simulink model "TST_RmtAPP_DD2"  (R2016b)
settings: Solver=FixedStepDiscrete  StartTime=0.0  StopTime=simTime  FixedStep=sampleTime  RelTol=1e-3
values from neighbouring files (symbols this model uses):
  testCase = 1    [initTST_RmtAPP_DD2_001.m]    (also in initTST_RmtAPP_DD2_002.m = 2)
libraries: simulink x13, UnitTest_Lib x10
settings Model: Creator=bianxuyin  LastModifiedBy=bianxuyin
settings DebuggingCC: SignalRangeChecking=error

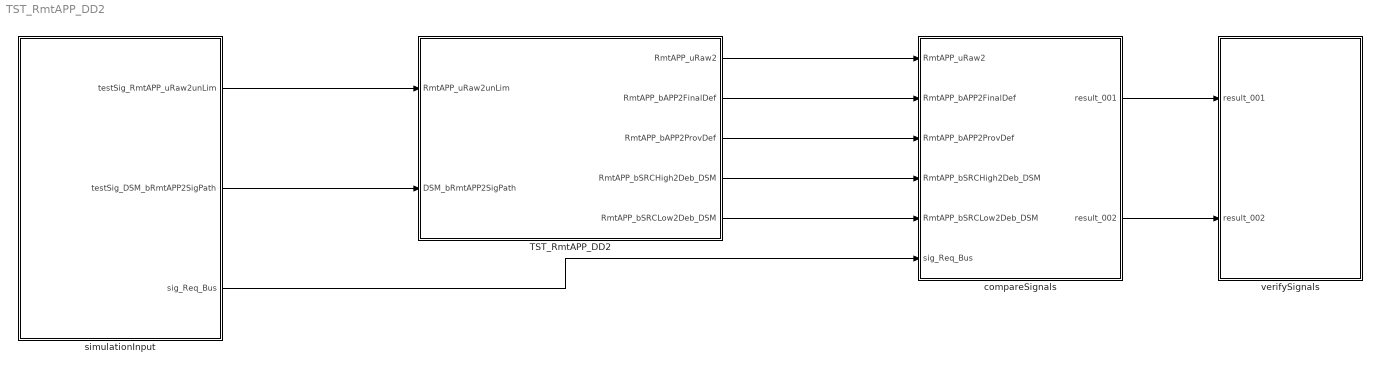
== system TST_RmtAPP_DD2 ==
  TST_RmtAPP_DD2 : Subsystem
  compareSignals : Subsystem
  simulationInput : Subsystem
  verifySignals : Subsystem
  wires:
  simulationInput/1(testSig_RmtAPP_uRaw2unLim) -> TST_RmtAPP_DD2/1(RmtAPP_uRaw2unLim)
  simulationInput/2(testSig_DSM_bRmtAPP2SigPath) -> TST_RmtAPP_DD2/2(DSM_bRmtAPP2SigPath)
  TST_RmtAPP_DD2/1(RmtAPP_uRaw2) -> compareSignals/1(RmtAPP_uRaw2)
  TST_RmtAPP_DD2/2(RmtAPP_bAPP2FinalDef) -> compareSignals/2(RmtAPP_bAPP2FinalDef)
  TST_RmtAPP_DD2/3(RmtAPP_bAPP2ProvDef) -> compareSignals/3(RmtAPP_bAPP2ProvDef)
  TST_RmtAPP_DD2/4(RmtAPP_bSRCHigh2Deb_DSM) -> compareSignals/4(RmtAPP_bSRCHigh2Deb_DSM)
  TST_RmtAPP_DD2/5(RmtAPP_bSRCLow2Deb_DSM) -> compareSignals/5(RmtAPP_bSRCLow2Deb_DSM)
  simulationInput/3(sig_Req_Bus) -> compareSignals/6(sig_Req_Bus)
  compareSignals/1(result_001) -> verifySignals/1(result_001)
  compareSignals/2(result_002) -> verifySignals/2(result_002)

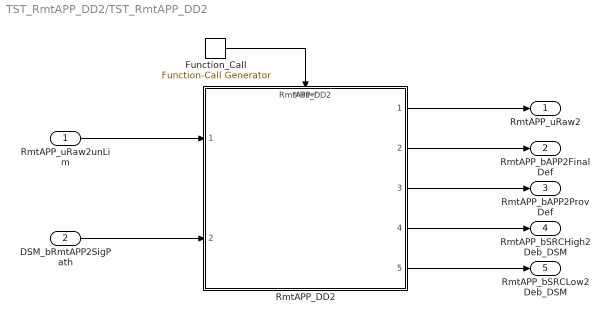
== system TST_RmtAPP_DD2/TST_RmtAPP_DD2 ==
  RmtAPP_uRaw2unLim : Inport
  DSM_bRmtAPP2SigPath : Inport  Port=2
  Function_Call : simulink/Ports & Subsystems/Function-Call Generator  sample_time=sampleTime  numberOfIterations=1
  RmtAPP_DD2 : ModelReference  ModelNameDialog=RmtAPP_DD2  SimulationMode=Normal  ModelReferenceVersion=1.5  TriggerPortName=function  TriggerPortTriggerType=function-call  TriggerPortStatesWhenEnabling=held
  RmtAPP_uRaw2 : Outport
  RmtAPP_bAPP2FinalDef : Outport  Port=2
  RmtAPP_bAPP2ProvDef : Outport  Port=3
  RmtAPP_bSRCHigh2Deb_DSM : Outport  Port=4
  RmtAPP_bSRCLow2Deb_DSM : Outport  Port=5
  wires:
  Function_Call/1 -> RmtAPP_DD2/Trigger
  RmtAPP_uRaw2unLim/1 -> RmtAPP_DD2/1
  DSM_bRmtAPP2SigPath/1 -> RmtAPP_DD2/2
  RmtAPP_DD2/1 -> RmtAPP_uRaw2/1
  RmtAPP_DD2/2 -> RmtAPP_bAPP2FinalDef/1
  RmtAPP_DD2/3 -> RmtAPP_bAPP2ProvDef/1
  RmtAPP_DD2/4 -> RmtAPP_bSRCHigh2Deb_DSM/1
  RmtAPP_DD2/5 -> RmtAPP_bSRCLow2Deb_DSM/1

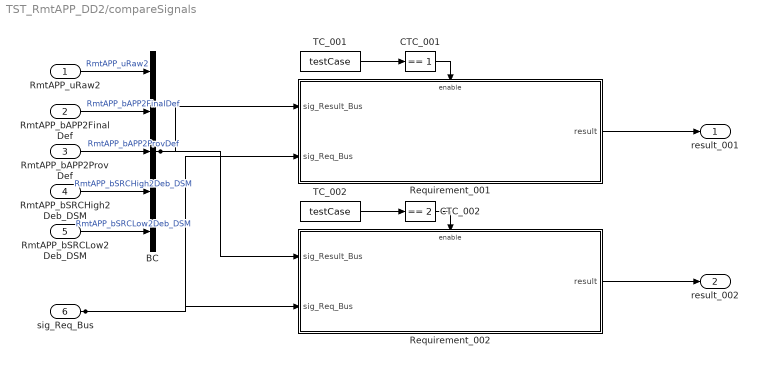
== system TST_RmtAPP_DD2/compareSignals ==
  RmtAPP_uRaw2 : Inport
  RmtAPP_bAPP2FinalDef : Inport  Port=2
  RmtAPP_bAPP2ProvDef : Inport  Port=3
  RmtAPP_bSRCHigh2Deb_DSM : Inport  Port=4
  RmtAPP_bSRCLow2Deb_DSM : Inport  Port=5
  sig_Req_Bus : Inport  Port=6
  BC : BusCreator  Inputs=5
  CTC_001 : simulink/Logic and Bit Operations/Compare To Constant  relop===  const=1  OutDataTypeStr=boolean
  CTC_002 : simulink/Logic and Bit Operations/Compare To Constant  relop===  const=2  OutDataTypeStr=boolean
  Requirement_001 : Subsystem
  Requirement_002 : Subsystem
  TC_001 : Constant  Value=testCase
  TC_002 : Constant  Value=testCase
  result_001 : Outport
  result_002 : Outport  Port=2
  wires:
  RmtAPP_uRaw2/1 -> BC/1  "RmtAPP_uRaw2"
  RmtAPP_bAPP2FinalDef/1 -> BC/2  "RmtAPP_bAPP2FinalDef"
  RmtAPP_bAPP2ProvDef/1 -> BC/3  "RmtAPP_bAPP2ProvDef"
  RmtAPP_bSRCHigh2Deb_DSM/1 -> BC/4  "RmtAPP_bSRCHigh2Deb_DSM"
  RmtAPP_bSRCLow2Deb_DSM/1 -> BC/5  "RmtAPP_bSRCLow2Deb_DSM"
  TC_001/1 -> CTC_001/1
  CTC_001/1 -> Requirement_001/Enable
  sig_Req_Bus/1 -> Requirement_001/2(sig_Req_Bus), Requirement_002/2(sig_Req_Bus)
  BC/1 -> Requirement_001/1(sig_Result_Bus), Requirement_002/1(sig_Result_Bus)
  Requirement_001/1(result) -> result_001/1
  TC_002/1 -> CTC_002/1
  CTC_002/1 -> Requirement_002/Enable
  Requirement_002/1(result) -> result_002/1

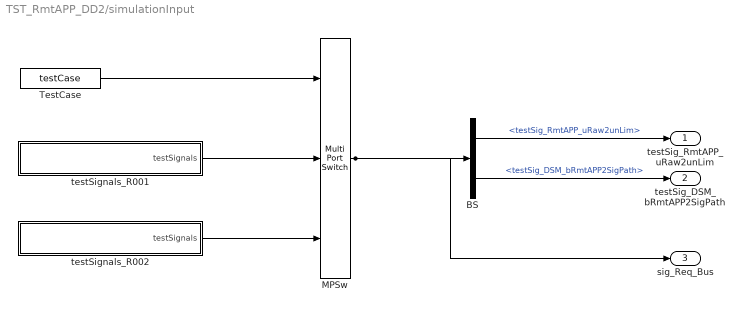
== system TST_RmtAPP_DD2/simulationInput ==
  BS : BusSelector  OutputSignals=testSig_RmtAPP_uRaw2unLim,testSig_DSM_bRmtAPP2SigPath
  MPSw : MultiPortSwitch  Inputs=2  SaturateOnIntegerOverflow=on  InputSameDT=on
  TestCase : Constant  Value=testCase
  testSignals_R001 : Subsystem
  testSignals_R002 : Subsystem
  testSig_RmtAPP_uRaw2unLim : Outport
  testSig_DSM_bRmtAPP2SigPath : Outport  Port=2
  sig_Req_Bus : Outport  Port=3
  wires:
  BS/1 -> testSig_RmtAPP_uRaw2unLim/1  "<testSig_RmtAPP_uRaw2unLim>"
  BS/2 -> testSig_DSM_bRmtAPP2SigPath/1  "<testSig_DSM_bRmtAPP2SigPath>"
  MPSw/1 -> BS/1, sig_Req_Bus/1
  TestCase/1 -> MPSw/1
  testSignals_R001/1(testSignals) -> MPSw/2
  testSignals_R002/1(testSignals) -> MPSw/3

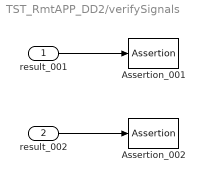
== system TST_RmtAPP_DD2/verifySignals ==
  result_001 : Inport
  result_002 : Inport  Port=2
  Assertion_001 : Assertion  Enabled=off
  Assertion_002 : Assertion  Enabled=off
  wires:
  result_001/1 -> Assertion_001/1
  result_002/1 -> Assertion_002/1

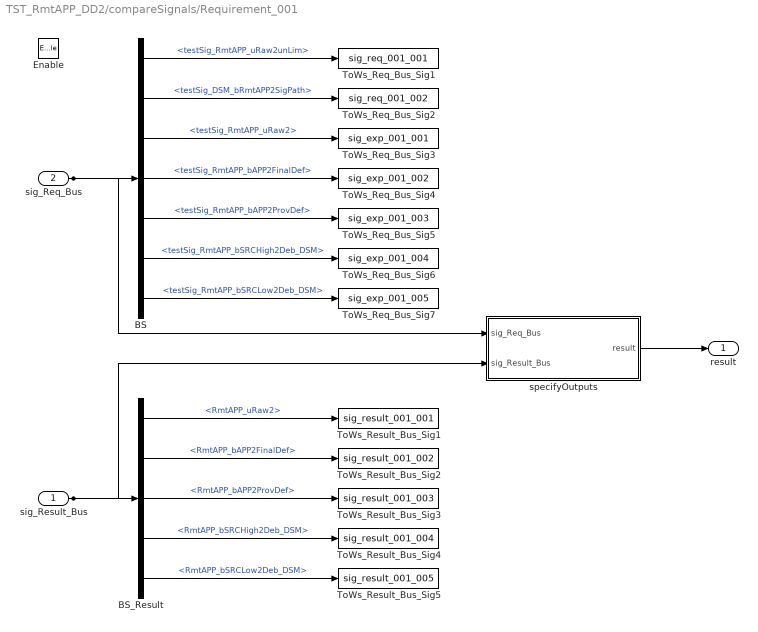
== system TST_RmtAPP_DD2/compareSignals/Requirement_001 ==
  sig_Result_Bus : Inport
  sig_Req_Bus : Inport  Port=2
  Enable : EnablePort
  BS : BusSelector  OutputSignals=testSig_RmtAPP_uRaw2unLim,testSig_DSM_bRmtAPP2SigPath,testSig_RmtAPP_uRaw2,testSig_RmtAPP_bAPP2FinalDef,testSig_RmtAPP_bAPP2ProvDef,testSig_RmtAPP_bSRCHigh2Deb_DSM,testSig_RmtAPP_bSRCLow2Deb_DSM
  BS_Result : BusSelector  OutputSignals=RmtAPP_uRaw2,RmtAPP_bAPP2FinalDef,RmtAPP_bAPP2ProvDef,RmtAPP_bSRCHigh2Deb_DSM,RmtAPP_bSRCLow2Deb_DSM
  ToWs_Req_Bus_Sig1 : ToWorkspace  VariableName=sig_req_001_001  SaveFormat=Structure With Time
  ToWs_Req_Bus_Sig2 : ToWorkspace  VariableName=sig_req_001_002  SaveFormat=Structure With Time
  ToWs_Req_Bus_Sig3 : ToWorkspace  VariableName=sig_exp_001_001  SaveFormat=Structure With Time
  ToWs_Req_Bus_Sig4 : ToWorkspace  VariableName=sig_exp_001_002  SaveFormat=Structure With Time
  ToWs_Req_Bus_Sig5 : ToWorkspace  VariableName=sig_exp_001_003  SaveFormat=Structure With Time
  ToWs_Req_Bus_Sig6 : ToWorkspace  VariableName=sig_exp_001_004  SaveFormat=Structure With Time
  ToWs_Req_Bus_Sig7 : ToWorkspace  VariableName=sig_exp_001_005  SaveFormat=Structure With Time
  ToWs_Result_Bus_Sig1 : ToWorkspace  VariableName=sig_result_001_001  SaveFormat=Structure With Time
  ToWs_Result_Bus_Sig2 : ToWorkspace  VariableName=sig_result_001_002  SaveFormat=Structure With Time
  ToWs_Result_Bus_Sig3 : ToWorkspace  VariableName=sig_result_001_003  SaveFormat=Structure With Time
  ToWs_Result_Bus_Sig4 : ToWorkspace  VariableName=sig_result_001_004  SaveFormat=Structure With Time
  ToWs_Result_Bus_Sig5 : ToWorkspace  VariableName=sig_result_001_005  SaveFormat=Structure With Time
  specifyOutputs : Subsystem
  result : Outport
  wires:
  sig_Req_Bus/1 -> BS/1, specifyOutputs/1(sig_Req_Bus)
  BS/1 -> ToWs_Req_Bus_Sig1/1  "<testSig_RmtAPP_uRaw2unLim>"
  BS/2 -> ToWs_Req_Bus_Sig2/1  "<testSig_DSM_bRmtAPP2SigPath>"
  BS/3 -> ToWs_Req_Bus_Sig3/1  "<testSig_RmtAPP_uRaw2>"
  BS/4 -> ToWs_Req_Bus_Sig4/1  "<testSig_RmtAPP_bAPP2FinalDef>"
  BS/5 -> ToWs_Req_Bus_Sig5/1  "<testSig_RmtAPP_bAPP2ProvDef>"
  BS/6 -> ToWs_Req_Bus_Sig6/1  "<testSig_RmtAPP_bSRCHigh2Deb_DSM>"
  BS/7 -> ToWs_Req_Bus_Sig7/1  "<testSig_RmtAPP_bSRCLow2Deb_DSM>"
  sig_Result_Bus/1 -> BS_Result/1, specifyOutputs/2(sig_Result_Bus)
  BS_Result/1 -> ToWs_Result_Bus_Sig1/1  "<RmtAPP_uRaw2>"
  BS_Result/2 -> ToWs_Result_Bus_Sig2/1  "<RmtAPP_bAPP2FinalDef>"
  BS_Result/3 -> ToWs_Result_Bus_Sig3/1  "<RmtAPP_bAPP2ProvDef>"
  BS_Result/4 -> ToWs_Result_Bus_Sig4/1  "<RmtAPP_bSRCHigh2Deb_DSM>"
  BS_Result/5 -> ToWs_Result_Bus_Sig5/1  "<RmtAPP_bSRCLow2Deb_DSM>"
  specifyOutputs/1(result) -> result/1

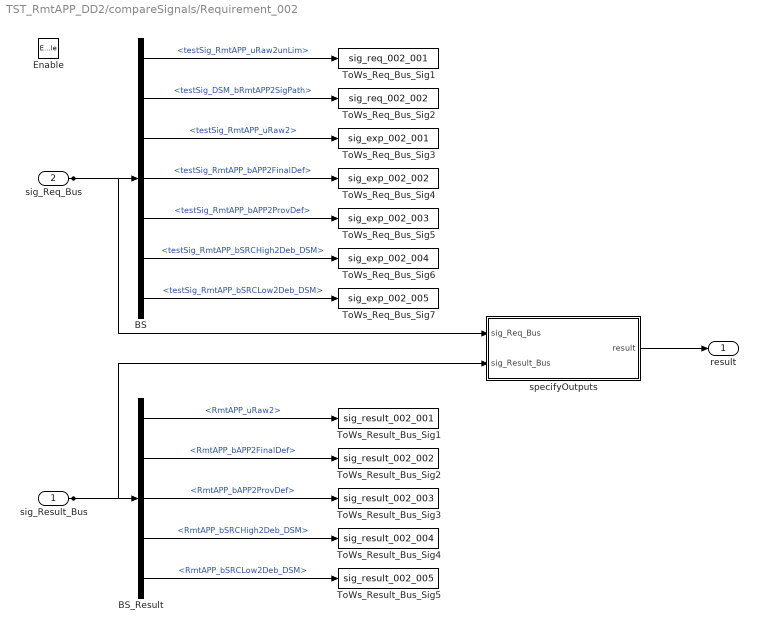
== system TST_RmtAPP_DD2/compareSignals/Requirement_002 ==
  sig_Result_Bus : Inport
  sig_Req_Bus : Inport  Port=2
  Enable : EnablePort
  BS : BusSelector  OutputSignals=testSig_RmtAPP_uRaw2unLim,testSig_DSM_bRmtAPP2SigPath,testSig_RmtAPP_uRaw2,testSig_RmtAPP_bAPP2FinalDef,testSig_RmtAPP_bAPP2ProvDef,testSig_RmtAPP_bSRCHigh2Deb_DSM,testSig_RmtAPP_bSRCLow2Deb_DSM
  BS_Result : BusSelector  OutputSignals=RmtAPP_uRaw2,RmtAPP_bAPP2FinalDef,RmtAPP_bAPP2ProvDef,RmtAPP_bSRCHigh2Deb_DSM,RmtAPP_bSRCLow2Deb_DSM
  ToWs_Req_Bus_Sig1 : ToWorkspace  VariableName=sig_req_002_001  SaveFormat=Structure With Time
  ToWs_Req_Bus_Sig2 : ToWorkspace  VariableName=sig_req_002_002  SaveFormat=Structure With Time
  ToWs_Req_Bus_Sig3 : ToWorkspace  VariableName=sig_exp_002_001  SaveFormat=Structure With Time
  ToWs_Req_Bus_Sig4 : ToWorkspace  VariableName=sig_exp_002_002  SaveFormat=Structure With Time
  ToWs_Req_Bus_Sig5 : ToWorkspace  VariableName=sig_exp_002_003  SaveFormat=Structure With Time
  ToWs_Req_Bus_Sig6 : ToWorkspace  VariableName=sig_exp_002_004  SaveFormat=Structure With Time
  ToWs_Req_Bus_Sig7 : ToWorkspace  VariableName=sig_exp_002_005  SaveFormat=Structure With Time
  ToWs_Result_Bus_Sig1 : ToWorkspace  VariableName=sig_result_002_001  SaveFormat=Structure With Time
  ToWs_Result_Bus_Sig2 : ToWorkspace  VariableName=sig_result_002_002  SaveFormat=Structure With Time
  ToWs_Result_Bus_Sig3 : ToWorkspace  VariableName=sig_result_002_003  SaveFormat=Structure With Time
  ToWs_Result_Bus_Sig4 : ToWorkspace  VariableName=sig_result_002_004  SaveFormat=Structure With Time
  ToWs_Result_Bus_Sig5 : ToWorkspace  VariableName=sig_result_002_005  SaveFormat=Structure With Time
  specifyOutputs : Subsystem
  result : Outport
  wires:
  sig_Req_Bus/1 -> BS/1, specifyOutputs/1(sig_Req_Bus)
  BS/1 -> ToWs_Req_Bus_Sig1/1  "<testSig_RmtAPP_uRaw2unLim>"
  BS/2 -> ToWs_Req_Bus_Sig2/1  "<testSig_DSM_bRmtAPP2SigPath>"
  BS/3 -> ToWs_Req_Bus_Sig3/1  "<testSig_RmtAPP_uRaw2>"
  BS/4 -> ToWs_Req_Bus_Sig4/1  "<testSig_RmtAPP_bAPP2FinalDef>"
  BS/5 -> ToWs_Req_Bus_Sig5/1  "<testSig_RmtAPP_bAPP2ProvDef>"
  BS/6 -> ToWs_Req_Bus_Sig6/1  "<testSig_RmtAPP_bSRCHigh2Deb_DSM>"
  BS/7 -> ToWs_Req_Bus_Sig7/1  "<testSig_RmtAPP_bSRCLow2Deb_DSM>"
  sig_Result_Bus/1 -> BS_Result/1, specifyOutputs/2(sig_Result_Bus)
  BS_Result/1 -> ToWs_Result_Bus_Sig1/1  "<RmtAPP_uRaw2>"
  BS_Result/2 -> ToWs_Result_Bus_Sig2/1  "<RmtAPP_bAPP2FinalDef>"
  BS_Result/3 -> ToWs_Result_Bus_Sig3/1  "<RmtAPP_bAPP2ProvDef>"
  BS_Result/4 -> ToWs_Result_Bus_Sig4/1  "<RmtAPP_bSRCHigh2Deb_DSM>"
  BS_Result/5 -> ToWs_Result_Bus_Sig5/1  "<RmtAPP_bSRCLow2Deb_DSM>"
  specifyOutputs/1(result) -> result/1

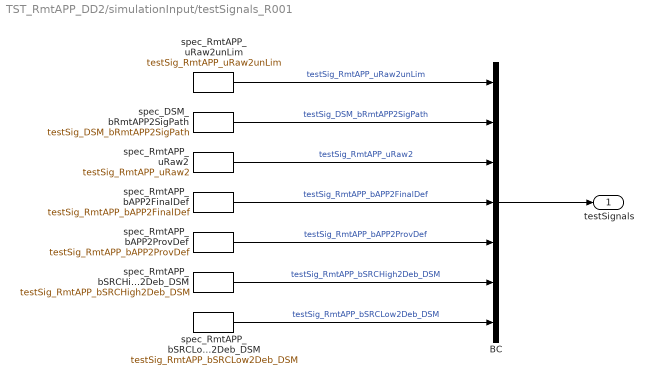
== system TST_RmtAPP_DD2/simulationInput/testSignals_R001 ==
  BC : BusCreator  Inputs=7
  spec_DSM_bRmtAPP2SigPath : FromWorkspace  VariableName=testSig_DSM_bRmtAPP2SigPath  Interpolate=off  OutputAfterFinalValue=Holding final value
  spec_RmtAPP_bAPP2FinalDef : FromWorkspace  VariableName=testSig_RmtAPP_bAPP2FinalDef  Interpolate=off  OutputAfterFinalValue=Holding final value
  spec_RmtAPP_bAPP2ProvDef : FromWorkspace  VariableName=testSig_RmtAPP_bAPP2ProvDef  Interpolate=off  OutputAfterFinalValue=Holding final value
  spec_RmtAPP_bSRCHigh2Deb_DSM : FromWorkspace  VariableName=testSig_RmtAPP_bSRCHigh2Deb_DSM  Interpolate=off  OutputAfterFinalValue=Holding final value
  spec_RmtAPP_bSRCLow2Deb_DSM : FromWorkspace  VariableName=testSig_RmtAPP_bSRCLow2Deb_DSM  Interpolate=off  OutputAfterFinalValue=Holding final value
  spec_RmtAPP_uRaw2 : FromWorkspace  VariableName=testSig_RmtAPP_uRaw2  Interpolate=off  OutputAfterFinalValue=Holding final value
  spec_RmtAPP_uRaw2unLim : FromWorkspace  VariableName=testSig_RmtAPP_uRaw2unLim  Interpolate=off  OutputAfterFinalValue=Holding final value
  testSignals : Outport
  wires:
  BC/1 -> testSignals/1
  spec_RmtAPP_uRaw2unLim/1 -> BC/1  "testSig_RmtAPP_uRaw2unLim"
  spec_DSM_bRmtAPP2SigPath/1 -> BC/2  "testSig_DSM_bRmtAPP2SigPath"
  spec_RmtAPP_uRaw2/1 -> BC/3  "testSig_RmtAPP_uRaw2"
  spec_RmtAPP_bAPP2FinalDef/1 -> BC/4  "testSig_RmtAPP_bAPP2FinalDef"
  spec_RmtAPP_bAPP2ProvDef/1 -> BC/5  "testSig_RmtAPP_bAPP2ProvDef"
  spec_RmtAPP_bSRCHigh2Deb_DSM/1 -> BC/6  "testSig_RmtAPP_bSRCHigh2Deb_DSM"
  spec_RmtAPP_bSRCLow2Deb_DSM/1 -> BC/7  "testSig_RmtAPP_bSRCLow2Deb_DSM"

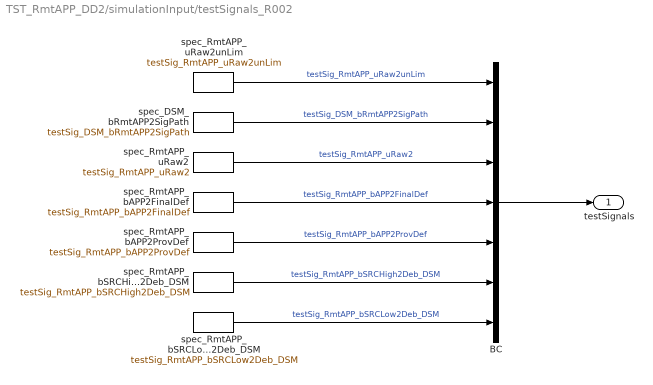
== system TST_RmtAPP_DD2/simulationInput/testSignals_R002 ==
  BC : BusCreator  Inputs=7
  spec_DSM_bRmtAPP2SigPath : FromWorkspace  VariableName=testSig_DSM_bRmtAPP2SigPath  Interpolate=off  OutputAfterFinalValue=Holding final value
  spec_RmtAPP_bAPP2FinalDef : FromWorkspace  VariableName=testSig_RmtAPP_bAPP2FinalDef  Interpolate=off  OutputAfterFinalValue=Holding final value
  spec_RmtAPP_bAPP2ProvDef : FromWorkspace  VariableName=testSig_RmtAPP_bAPP2ProvDef  Interpolate=off  OutputAfterFinalValue=Holding final value
  spec_RmtAPP_bSRCHigh2Deb_DSM : FromWorkspace  VariableName=testSig_RmtAPP_bSRCHigh2Deb_DSM  Interpolate=off  OutputAfterFinalValue=Holding final value
  spec_RmtAPP_bSRCLow2Deb_DSM : FromWorkspace  VariableName=testSig_RmtAPP_bSRCLow2Deb_DSM  Interpolate=off  OutputAfterFinalValue=Holding final value
  spec_RmtAPP_uRaw2 : FromWorkspace  VariableName=testSig_RmtAPP_uRaw2  Interpolate=off  OutputAfterFinalValue=Holding final value
  spec_RmtAPP_uRaw2unLim : FromWorkspace  VariableName=testSig_RmtAPP_uRaw2unLim  Interpolate=off  OutputAfterFinalValue=Holding final value
  testSignals : Outport
  wires:
  BC/1 -> testSignals/1
  spec_RmtAPP_uRaw2unLim/1 -> BC/1  "testSig_RmtAPP_uRaw2unLim"
  spec_DSM_bRmtAPP2SigPath/1 -> BC/2  "testSig_DSM_bRmtAPP2SigPath"
  spec_RmtAPP_uRaw2/1 -> BC/3  "testSig_RmtAPP_uRaw2"
  spec_RmtAPP_bAPP2FinalDef/1 -> BC/4  "testSig_RmtAPP_bAPP2FinalDef"
  spec_RmtAPP_bAPP2ProvDef/1 -> BC/5  "testSig_RmtAPP_bAPP2ProvDef"
  spec_RmtAPP_bSRCHigh2Deb_DSM/1 -> BC/6  "testSig_RmtAPP_bSRCHigh2Deb_DSM"
  spec_RmtAPP_bSRCLow2Deb_DSM/1 -> BC/7  "testSig_RmtAPP_bSRCLow2Deb_DSM"

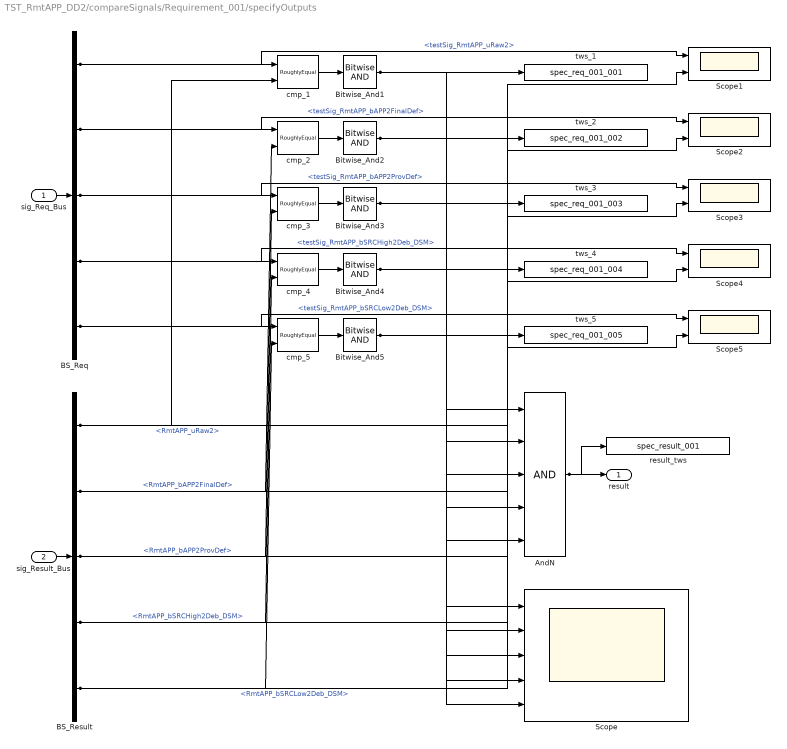
== system TST_RmtAPP_DD2/compareSignals/Requirement_001/specifyOutputs ==
  sig_Req_Bus : Inport
  sig_Result_Bus : Inport  Port=2
  AndN : Logic  Inputs=5
  BS_Req : BusSelector  OutputSignals=testSig_RmtAPP_uRaw2,testSig_RmtAPP_bAPP2FinalDef,testSig_RmtAPP_bAPP2ProvDef,testSig_RmtAPP_bSRCHigh2Deb_DSM,testSig_RmtAPP_bSRCLow2Deb_DSM
  BS_Result : BusSelector  OutputSignals=RmtAPP_uRaw2,RmtAPP_bAPP2FinalDef,RmtAPP_bAPP2ProvDef,RmtAPP_bSRCHigh2Deb_DSM,RmtAPP_bSRCLow2Deb_DSM
  Bitwise_And{1..5} (5 alike) : simulink/Logic and Bit Operations/Bitwise Operator  logicop=AND  UseBitMask=off  BitMask=bin2dec('11011001')  BitMaskRealWorld=Stored Integer
  Scope : Scope  NumInputPorts=5
  Scope{1..5} (5 alike) : Scope  NumInputPorts=2
  cmp_{1..5} (5 alike) : UnitTest_Lib/RoughlyEqual  slope=0.1
  result_tws : ToWorkspace  VariableName=spec_result_001
  tws_1 : ToWorkspace  VariableName=spec_req_001_001
  tws_2 : ToWorkspace  VariableName=spec_req_001_002
  tws_3 : ToWorkspace  VariableName=spec_req_001_003
  tws_4 : ToWorkspace  VariableName=spec_req_001_004
  tws_5 : ToWorkspace  VariableName=spec_req_001_005
  result : Outport
  wires:
  sig_Req_Bus/1 -> BS_Req/1
  sig_Result_Bus/1 -> BS_Result/1
  AndN/1 -> result/1, result_tws/1
  BS_Req/1 -> cmp_1/1, Scope1/1  "<testSig_RmtAPP_uRaw2>"
  BS_Result/1 -> cmp_1/2, Scope1/2  "<RmtAPP_uRaw2>"
  cmp_1/1 -> Bitwise_And1/1
  Bitwise_And1/1 -> tws_1/1, AndN/1, Scope/1
  BS_Req/2 -> cmp_2/1, Scope2/1  "<testSig_RmtAPP_bAPP2FinalDef>"
  BS_Result/2 -> cmp_2/2, Scope2/2  "<RmtAPP_bAPP2FinalDef>"
  cmp_2/1 -> Bitwise_And2/1
  Bitwise_And2/1 -> tws_2/1, AndN/2, Scope/2
  BS_Req/3 -> cmp_3/1, Scope3/1  "<testSig_RmtAPP_bAPP2ProvDef>"
  BS_Result/3 -> cmp_3/2, Scope3/2  "<RmtAPP_bAPP2ProvDef>"
  cmp_3/1 -> Bitwise_And3/1
  Bitwise_And3/1 -> tws_3/1, AndN/3, Scope/3
  BS_Req/4 -> cmp_4/1, Scope4/1  "<testSig_RmtAPP_bSRCHigh2Deb_DSM>"
  BS_Result/4 -> cmp_4/2, Scope4/2  "<RmtAPP_bSRCHigh2Deb_DSM>"
  cmp_4/1 -> Bitwise_And4/1
  Bitwise_And4/1 -> tws_4/1, AndN/4, Scope/4
  BS_Req/5 -> cmp_5/1, Scope5/1  "<testSig_RmtAPP_bSRCLow2Deb_DSM>"
  BS_Result/5 -> cmp_5/2, Scope5/2  "<RmtAPP_bSRCLow2Deb_DSM>"
  cmp_5/1 -> Bitwise_And5/1
  Bitwise_And5/1 -> tws_5/1, AndN/5, Scope/5

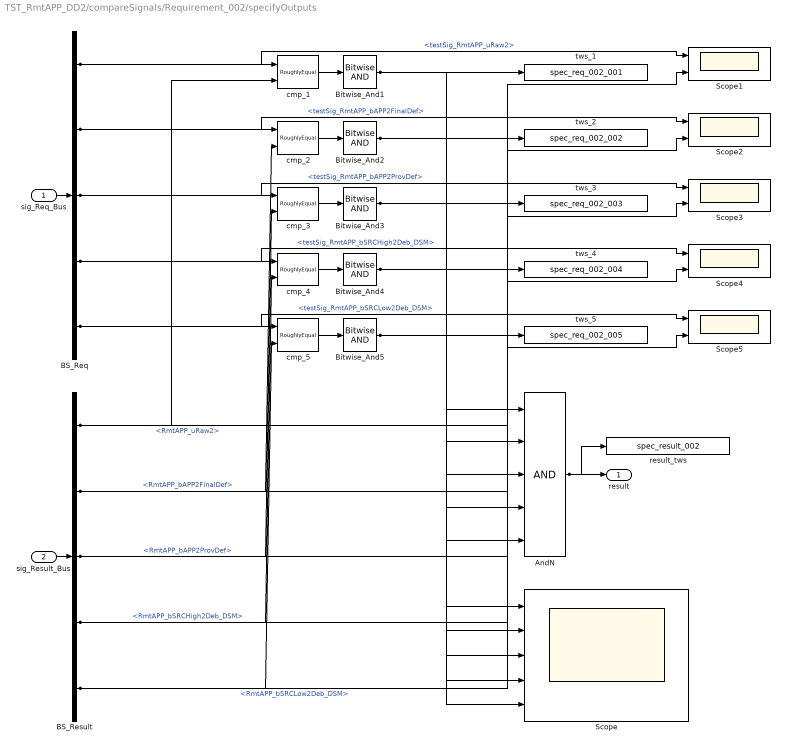
== system TST_RmtAPP_DD2/compareSignals/Requirement_002/specifyOutputs ==
  sig_Req_Bus : Inport
  sig_Result_Bus : Inport  Port=2
  AndN : Logic  Inputs=5
  BS_Req : BusSelector  OutputSignals=testSig_RmtAPP_uRaw2,testSig_RmtAPP_bAPP2FinalDef,testSig_RmtAPP_bAPP2ProvDef,testSig_RmtAPP_bSRCHigh2Deb_DSM,testSig_RmtAPP_bSRCLow2Deb_DSM
  BS_Result : BusSelector  OutputSignals=RmtAPP_uRaw2,RmtAPP_bAPP2FinalDef,RmtAPP_bAPP2ProvDef,RmtAPP_bSRCHigh2Deb_DSM,RmtAPP_bSRCLow2Deb_DSM
  Bitwise_And{1..5} (5 alike) : simulink/Logic and Bit Operations/Bitwise Operator  logicop=AND  UseBitMask=off  BitMask=bin2dec('11011001')  BitMaskRealWorld=Stored Integer
  Scope : Scope  NumInputPorts=5
  Scope{1..5} (5 alike) : Scope  NumInputPorts=2
  cmp_{1..5} (5 alike) : UnitTest_Lib/RoughlyEqual  slope=0.1
  result_tws : ToWorkspace  VariableName=spec_result_002
  tws_1 : ToWorkspace  VariableName=spec_req_002_001
  tws_2 : ToWorkspace  VariableName=spec_req_002_002
  tws_3 : ToWorkspace  VariableName=spec_req_002_003
  tws_4 : ToWorkspace  VariableName=spec_req_002_004
  tws_5 : ToWorkspace  VariableName=spec_req_002_005
  result : Outport
  wires:
  sig_Req_Bus/1 -> BS_Req/1
  sig_Result_Bus/1 -> BS_Result/1
  AndN/1 -> result/1, result_tws/1
  BS_Req/1 -> cmp_1/1, Scope1/1  "<testSig_RmtAPP_uRaw2>"
  BS_Result/1 -> cmp_1/2, Scope1/2  "<RmtAPP_uRaw2>"
  cmp_1/1 -> Bitwise_And1/1
  Bitwise_And1/1 -> tws_1/1, AndN/1, Scope/1
  BS_Req/2 -> cmp_2/1, Scope2/1  "<testSig_RmtAPP_bAPP2FinalDef>"
  BS_Result/2 -> cmp_2/2, Scope2/2  "<RmtAPP_bAPP2FinalDef>"
  cmp_2/1 -> Bitwise_And2/1
  Bitwise_And2/1 -> tws_2/1, AndN/2, Scope/2
  BS_Req/3 -> cmp_3/1, Scope3/1  "<testSig_RmtAPP_bAPP2ProvDef>"
  BS_Result/3 -> cmp_3/2, Scope3/2  "<RmtAPP_bAPP2ProvDef>"
  cmp_3/1 -> Bitwise_And3/1
  Bitwise_And3/1 -> tws_3/1, AndN/3, Scope/3
  BS_Req/4 -> cmp_4/1, Scope4/1  "<testSig_RmtAPP_bSRCHigh2Deb_DSM>"
  BS_Result/4 -> cmp_4/2, Scope4/2  "<RmtAPP_bSRCHigh2Deb_DSM>"
  cmp_4/1 -> Bitwise_And4/1
  Bitwise_And4/1 -> tws_4/1, AndN/4, Scope/4
  BS_Req/5 -> cmp_5/1, Scope5/1  "<testSig_RmtAPP_bSRCLow2Deb_DSM>"
  BS_Result/5 -> cmp_5/2, Scope5/2  "<RmtAPP_bSRCLow2Deb_DSM>"
  cmp_5/1 -> Bitwise_And5/1
  Bitwise_And5/1 -> tws_5/1, AndN/5, Scope/5
